simulink model "Demo_MatrixSign_cs"  (Simulink 7.6)
settings: Solver=FixedStepDiscrete  SolverMode=SingleTasking  StartTime=0.0  StopTime=10  FixedStep=1/20  RelTol=1e-3
model workspace (MAT data in the model file):
  mbox_table.block_array(1).src = 'built-in/Subsystem'
  mbox_table.block_array(1).dest = 'Demo_MatrixSign_cs/HighwayOverhang_1'
  mbox_table.block_array(1).mode = 0
  mbox_table.block_array(2).src = 'simulink/Sinks/Out1'
  mbox_table.block_array(2).dest = 'Demo_MatrixSign_cs/HighwayOverhang_1/VISUMatrixSign_HighwayOverhang_1'
  mbox_table.block_array(2).mode = 0
  mbox_table.block_array(3).src = 'PreScanSimulinkLibrary/VisuMatrixSign'
  mbox_table.block_array(3).dest = 'Demo_MatrixSign_cs/VISUMatrixSign_HighwayOverhang_1'
  mbox_table.block_array(3).mode = 0
  mbox_table.block_array(4).src = 'PreScanSimulinkLibrary/MuxMatrixSign'
  mbox_table.block_array(4).dest = 'Demo_MatrixSign_cs/HighwayOverhang_1/VISUMatrixSign_Mux'
  mbox_table.block_array(4).mode = 0
  mbox_table.block_array(5).src = 'simulink/Sources/Constant'
  mbox_table.block_array(5).dest = 'Demo_MatrixSign_cs/HighwayOverhang_1/VISUMatrixSign_Mux/MatrixSign_1_InitialResource'
  mbox_table.block_array(5).mode = 0
  mbox_table.block_array(6).src = 'simulink/Signal Routing/Switch'
  mbox_table.block_array(6).dest = 'Demo_MatrixSign_cs/HighwayOverhang_1/VISUMatrixSign_Mux/MatrixSign_1_Switch'
  mbox_table.block_array(6).mode = 0
  mbox_table.block_array(7).src = 'Demo_MatrixSign_cs/HighwayOverhang_1/VISUMatrixSign_Mux/MatrixSign_1'
  mbox_table.block_array(7).dest = 'Demo_MatrixSign_cs/HighwayOverhang_1/VISUMatrixSign_Mux/MatrixSign_2'
  mbox_table.block_array(7).mode = 0
  mbox_table.block_array(8).src = 'simulink/Sources/Constant'
  mbox_table.block_array(8).dest = 'Demo_MatrixSign_cs/HighwayOverhang_1/VISUMatrixSign_Mux/MatrixSign_2_InitialResource'
  mbox_table.block_array(8).mode = 0
  mbox_table.block_array(9).src = 'simulink/Signal Routing/Switch'
  mbox_table.block_array(9).dest = 'Demo_MatrixSign_cs/HighwayOverhang_1/VISUMatrixSign_Mux/MatrixSign_2_Switch'
  mbox_table.block_array(9).mode = 0
  mbox_table.block_array(10).src = 'Demo_MatrixSign_cs/VISUMatrixSign_HighwayOverhang_1/visu_MatrixSign_1'
  mbox_table.block_array(10).dest = 'Demo_MatrixSign_cs/VISUMatrixSign_HighwayOverhang_1/visu_MatrixSign_2'
  mbox_table.block_array(10).mode = 0
  mbox_table.block_array(11).src = 'built-in/Note'
  mbox_table.block_array(11).dest = 'Demo_MatrixSign_cs/HighwayOverhang_1/Resources     
    | 
    | 1: .\InformationSign\MatrixSign_Speed_50.png: MatrixSign_Speed_50
    | 2: .\InformationSign\MatrixSign_Speed_70.png: MatrixSign_Speed_70
    | 3: .\InformationSign\MatrixSign_Speed_End.png: MatrixSign_Speed_End
    | 4: .\InformationSign\MatrixSign_Empty.png: MatrixSign_Empty'
  mbox_table.block_array(11).mode = 0
  mbox_table.block_array(12).src = 'built-in/Note'
  mbox_table.block_array(12).dest = 'Demo_MatrixSign_cs/HighwayOverhang_1/Resources     '
  mbox_table.block_array(12).mode = 0
  mbox_table.block_array(13).src = 'simulink/Sinks/Out1'
  mbox_table.block_array(13).dest = 'Demo_MatrixSign_cs/HighwayOverhang_1/VISUMatrixSignLights_HighwayOverhang_1'
  mbox_table.block_array(13).mode = 0
  mbox_table.block_array(14).src = 'PreScanSimulinkLibrary/VisuMatrixSignLights'
  mbox_table.block_array(14).dest = 'Demo_MatrixSign_cs/VISUMatrixSignLights_HighwayOverhang_1'
  mbox_table.block_array(14).mode = 0
  mbox_table.block_array(15).src = 'PreScanSimulinkLibrary/MuxMatrixSignLights'
  mbox_table.block_array(15).dest = 'Demo_MatrixSign_cs/HighwayOverhang_1/VISUMatrixSignLights_Mux'
  mbox_table.block_array(15).mode = 0
  mbox_table.block_array(16).src = 'Demo_MatrixSign_cs/HighwayOverhang_1/VISUMatrixSignLights_Mux/MatrixSign_1'
  mbox_table.block_array(16).dest = 'Demo_MatrixSign_cs/HighwayOverhang_1/VISUMatrixSignLights_Mux/MatrixSign_2'
  mbox_table.block_array(16).mode = 0
  mbox_table.block_array(17).src = 'Demo_MatrixSign_cs/VISUMatrixSignLights_HighwayOverhang_1/conv_Orange_1'
  mbox_table.block_array(17).dest = 'Demo_MatrixSign_cs/VISUMatrixSignLights_HighwayOverhang_1/conv_Orange_2'
  mbox_table.block_array(17).mode = 0
  mbox_table.block_array(18).src = 'Demo_MatrixSign_cs/VISUMatrixSignLights_HighwayOverhang_1/visu_MatrixSignLights_1'
  mbox_table.block_array(18).dest = 'Demo_MatrixSign_cs/VISUMatrixSignLights_HighwayOverhang_1/visu_MatrixSignLights_2'
  mbox_table.block_array(18).mode = 0
  mbox_table.block_array(19).src = 'Demo_MatrixSign_cs/VISUMatrixSignLights_HighwayOverhang_1/conv_Orange_1'
  mbox_table.block_array(19).dest = 'Demo_MatrixSign_cs/VISUMatrixSignLights_HighwayOverhang_1/conv_Orange_3'
  mbox_table.block_array(19).mode = 0
  mbox_table.block_array(20).src = 'Demo_MatrixSign_cs/VISUMatrixSignLights_HighwayOverhang_1/visu_MatrixSignLights_1'
  mbox_table.block_array(20).dest = 'Demo_MatrixSign_cs/VISUMatrixSignLights_HighwayOverhang_1/visu_MatrixSignLights_3'
  mbox_table.block_array(20).mode = 0
  mbox_table.block_array(21).src = 'Demo_MatrixSign_cs/VISUMatrixSignLights_HighwayOverhang_1/conv_Orange_1'
  mbox_table.block_array(21).dest = 'Demo_MatrixSign_cs/VISUMatrixSignLights_HighwayOverhang_1/conv_Orange_4'
  mbox_table.block_array(21).mode = 0
  mbox_table.block_array(22).src = 'Demo_MatrixSign_cs/VISUMatrixSignLights_HighwayOverhang_1/visu_MatrixSignLights_1'
  mbox_table.block_array(22).dest = 'Demo_MatrixSign_cs/VISUMatrixSignLights_HighwayOverhang_1/visu_MatrixSignLights_4'
  mbox_table.block_array(22).mode = 0
  mbox_table.block_array(23).src = 'Demo_MatrixSign_cs/VISUMatrixSignLights_HighwayOverhang_1/conv_Orange_1'
  mbox_table.block_array(23).dest = 'Demo_MatrixSign_cs/VISUMatrixSignLights_HighwayOverhang_1/conv_Orange_5'
  mbox_table.block_array(23).mode = 0
  mbox_table.block_array(24).src = 'Demo_MatrixSign_cs/VISUMatrixSignLights_HighwayOverhang_1/visu_MatrixSignLights_1'
  mbox_table.block_array(24).dest = 'Demo_MatrixSign_cs/VISUMatrixSignLights_HighwayOverhang_1/visu_MatrixSignLights_5'
  mbox_table.block_array(24).mode = 0
  mbox_table.block_array(25).src = 'Demo_MatrixSign_cs/VISUMatrixSignLights_HighwayOverhang_1/conv_Orange_1'
  mbox_table.block_array(25).dest = 'Demo_MatrixSign_cs/VISUMatrixSignLights_HighwayOverhang_1/conv_Orange_6'
  mbox_table.block_array(25).mode = 0
  mbox_table.block_array(26).src = 'Demo_MatrixSign_cs/VISUMatrixSignLights_HighwayOverhang_1/visu_MatrixSignLights_1'
  mbox_table.block_array(26).dest = 'Demo_MatrixSign_cs/VISUMatrixSignLights_HighwayOverhang_1/visu_MatrixSignLights_6'
  mbox_table.block_array(26).mode = 0
  mbox_table.block_array(27).src = 'Demo_MatrixSign_cs/VISUMatrixSignLights_HighwayOverhang_1/conv_Orange_1'
  mbox_table.block_array(27).dest = 'Demo_MatrixSign_cs/VISUMatrixSignLights_HighwayOverhang_1/conv_Orange_7'
  mbox_table.block_array(27).mode = 0
  mbox_table.block_array(28).src = 'Demo_MatrixSign_cs/VISUMatrixSignLights_HighwayOverhang_1/visu_MatrixSignLights_1'
  mbox_table.block_array(28).dest = 'Demo_MatrixSign_cs/VISUMatrixSignLights_HighwayOverhang_1/visu_MatrixSignLights_7'
  mbox_table.block_array(28).mode = 0
  mbox_table.block_array(29).src = 'Demo_MatrixSign_cs/VISUMatrixSignLights_HighwayOverhang_1/conv_Orange_1'
  mbox_table.block_array(29).dest = 'Demo_MatrixSign_cs/VISUMatrixSignLights_HighwayOverhang_1/conv_Orange_8'
  mbox_table.block_array(29).mode = 0
  mbox_table.block_array(30).src = 'Demo_MatrixSign_cs/VISUMatrixSignLights_HighwayOverhang_1/visu_MatrixSignLights_1'
  mbox_table.block_array(30).dest = 'Demo_MatrixSign_cs/VISUMatrixSignLights_HighwayOverhang_1/visu_MatrixSignLights_8'
  mbox_table.block_array(30).mode = 0
  mbox_table.block_array(31).src = 'SimCoreLibrary/SimCoreConfiguration'
  mbox_table.block_array(31).dest = 'Demo_MatrixSign_cs/SimCoreConfiguration'
  mbox_table.block_array(31).mode = 0
  mbox_table.block_array(32).src = 'SimCoreLibrary/Actuators'
  mbox_table.block_array(32).dest = 'Demo_MatrixSign_cs/Actuators'
  mbox_table.block_array(32).mode = 0
  mbox_table.block_array(33).src = 'SimCoreLibrary/SetActuators'
  mbox_table.block_array(33).dest = 'Demo_MatrixSign_cs/SetActuators'
  mbox_table.block_array(33).mode = 0
  mbox_table.block_array(34).src = 'SimCoreLibrary/SimCoreInfo'
  mbox_table.block_array(34).dest = 'Demo_MatrixSign_cs/SimCoreInfo'
  mbox_table.block_array(34).mode = 0
  mbox_table.block_array(35).src = 'PreScanSimulinkLibrary/Regenerate'
  mbox_table.block_array(35).dest = 'Demo_MatrixSign_cs/Regenerate'
  mbox_table.block_array(35).mode = 0
  mbox_table.block_array(36).src = 'PreScanSimulinkLibrary/Record for Replay  '
  mbox_table.block_array(36).dest = 'Demo_MatrixSign_cs/Record for Replay  '
  mbox_table.block_array(36).mode = 0
  mbox_table.block_array(37).src = 'PreScanSimulinkLibrary/Open Useful Blocks'
  mbox_table.block_array(37).dest = 'Demo_MatrixSign_cs/Open Useful Blocks'
  mbox_table.block_array(37).mode = 0
  mbox_table.block_array(38).src = 'PreScanSimulinkLibrary/PreScan Options   '
  mbox_table.block_array(38).dest = 'Demo_MatrixSign_cs/PreScan Options   '
  mbox_table.block_array(38).mode = 0
  mbox_table.block_array(39).src = 'built-in/Note'
  mbox_table.block_array(39).dest = 'Demo_MatrixSign_cs/Version:                  '
  mbox_table.block_array(39).mode = 0
  mbox_table.block_array(40).src = 'built-in/Note'
  mbox_table.block_array(40).dest = 'Demo_MatrixSign_cs/7.4.0'
  mbox_table.block_array(40).mode = 0
  mbox_table.block_array(41).src = 'built-in/Note'
  mbox_table.block_array(41).dest = 'Demo_MatrixSign_cs/Author(s):                '
  mbox_table.block_array(41).mode = 0
  mbox_table.block_array(42).src = 'built-in/Note'
  mbox_table.block_array(42).dest = 'Demo_MatrixSign_cs/F.J.W. Leneman, (c) TNO 2008'
  mbox_table.block_array(42).mode = 0
  mbox_table.block_array(43).src = 'built-in/Note'
  mbox_table.block_array(43).dest = 'Demo_MatrixSign_cs/Descriptive text:      '
  mbox_table.block_array(43).mode = 0
  mbox_table.block_array(44).src = 'built-in/Note'
  mbox_table.block_array(44).dest = 'Demo_MatrixSign_cs/Demo MatrixSign
    | The demo illustrates the use of
    | the Matrix Sign.
    | 
    | Key-elements:
    | - Matrix Sign
    | - Overhang
    | - Signal Builder Block'
  mbox_table.block_array(44).mode = 0
  mbox_table.block_array(45).src = 'built-in/Note'
  mbox_table.block_array(45).dest = 'Demo_MatrixSign_cs/ID
    | 
    | 1'
  mbox_table.block_array(45).mode = 0
  mbox_table.block_array(46).src = 'built-in/Note'
  mbox_table.block_array(46).dest = 'Demo_MatrixSign_cs/OBU-Beacon ID
    | 
    | '
  mbox_table.block_array(46).mode = 0
  mbox_table.block_array(47).src = 'built-in/Note'
  mbox_table.block_array(47).dest = 'Demo_MatrixSign_cs/TypeID
    | 
    | 15'
  mbox_table.block_array(47).mode = 0
  mbox_table.block_array(48).src = 'built-in/Note'
  mbox_table.block_array(48).dest = 'Demo_MatrixSign_cs/TypeTag
    | 
    | Anim traffic sign'
  mbox_table.block_array(48).mode = 0
  mbox_table.block_array(49).src = 'built-in/Note'
  mbox_table.block_array(49).dest = 'Demo_MatrixSign_cs/SD
    | 
    | Y'
  mbox_table.block_array(49).mode = 0
  mbox_table.block_array(50).src = 'built-in/Note'
  mbox_table.block_array(50).dest = 'Demo_MatrixSign_cs/CD
    | 
    | N'
  mbox_table.block_array(50).mode = 0
  mbox_table.block_array(51).src = 'built-in/Note'
  mbox_table.block_array(51).dest = 'Demo_MatrixSign_cs/Name
    | 
    | HighwayOverhang_1'
  mbox_table.block_array(51).mode = 0
  mbox_table.block_array(52).src = 'built-in/Note'
  mbox_table.block_array(52).dest = 'Demo_MatrixSign_cs/Num ID       OBU-Beacon ID     Type ID      Type Tag             SD        CD             Name                          '
  mbox_table.block_array(52).mode = 0
  mbox_table.block_array(53).src = 'built-in/Terminator'
  mbox_table.block_array(53).dest = 'Demo_MatrixSign_cs/Terminator_1'
  mbox_table.block_array(53).mode = 1
  mbox_table.block_index : java.util.Hashtable (value not decoded)
  mbox_table.line_array(1).sys = 'Demo_MatrixSign_cs/HighwayOverhang_1'
  mbox_table.line_array(1).line_id = 'L1'
  mbox_table.line_array(1).iport = 'VISUMatrixSign_HighwayOverhang_1/1'
  mbox_table.line_array(1).oport = 'VISUMatrixSign_Mux/1'
  mbox_table.line_array(1).mode = 0
  mbox_table.line_array(2).sys = 'Demo_MatrixSign_cs'
  mbox_table.line_array(2).line_id = 'L2'
  mbox_table.line_array(2).iport = 'VISUMatrixSign_HighwayOverhang_1/1'
  mbox_table.line_array(2).oport = 'HighwayOverhang_1/1'
  mbox_table.line_array(2).mode = 0
  mbox_table.line_array(3).sys = 'Demo_MatrixSign_cs/HighwayOverhang_1/VISUMatrixSign_Mux'
  mbox_table.line_array(3).line_id = 'L4'
  mbox_table.line_array(3).iport = 'MatrixSign_1_Switch/1'
  mbox_table.line_array(3).oport = 'MatrixSign_1/1'
  mbox_table.line_array(3).mode = 0
  mbox_table.line_array(4).sys = 'Demo_MatrixSign_cs/HighwayOverhang_1/VISUMatrixSign_Mux'
  mbox_table.line_array(4).line_id = 'L4'
  mbox_table.line_array(4).iport = 'MatrixSign_1_Switch/2'
  mbox_table.line_array(4).oport = 'MatrixSign_1/1'
  mbox_table.line_array(4).mode = 0
  mbox_table.line_array(5).sys = 'Demo_MatrixSign_cs/HighwayOverhang_1/VISUMatrixSign_Mux'
  mbox_table.line_array(5).line_id = 'L5'
  mbox_table.line_array(5).iport = 'MatrixSign_1_Switch/3'
  mbox_table.line_array(5).oport = 'MatrixSign_1_InitialResource/1'
  mbox_table.line_array(5).mode = 0
  mbox_table.line_array(6).sys = 'Demo_MatrixSign_cs/HighwayOverhang_1/VISUMatrixSign_Mux'
  mbox_table.line_array(6).line_id = 'L6'
  mbox_table.line_array(6).iport = 'SubMuxMatrixSign/1'
  mbox_table.line_array(6).oport = 'MatrixSign_1_Switch/1'
  mbox_table.line_array(6).mode = 0
  mbox_table.line_array(7).sys = 'Demo_MatrixSign_cs/HighwayOverhang_1/VISUMatrixSign_Mux'
  mbox_table.line_array(7).line_id = 'L8'
  mbox_table.line_array(7).iport = 'MatrixSign_2_Switch/1'
  mbox_table.line_array(7).oport = 'MatrixSign_2/1'
  mbox_table.line_array(7).mode = 0
  mbox_table.line_array(8).sys = 'Demo_MatrixSign_cs/HighwayOverhang_1/VISUMatrixSign_Mux'
  mbox_table.line_array(8).line_id = 'L8'
  mbox_table.line_array(8).iport = 'MatrixSign_2_Switch/2'
  mbox_table.line_array(8).oport = 'MatrixSign_2/1'
  mbox_table.line_array(8).mode = 0
  mbox_table.line_array(9).sys = 'Demo_MatrixSign_cs/HighwayOverhang_1/VISUMatrixSign_Mux'
  mbox_table.line_array(9).line_id = 'L9'
  mbox_table.line_array(9).iport = 'MatrixSign_2_Switch/3'
  mbox_table.line_array(9).oport = 'MatrixSign_2_InitialResource/1'
  mbox_table.line_array(9).mode = 0
  mbox_table.line_array(10).sys = 'Demo_MatrixSign_cs/HighwayOverhang_1/VISUMatrixSign_Mux'
  mbox_table.line_array(10).line_id = 'L10'
  mbox_table.line_array(10).iport = 'SubMuxMatrixSign/2'
  mbox_table.line_array(10).oport = 'MatrixSign_2_Switch/1'
  mbox_table.line_array(10).mode = 0
  mbox_table.line_array(11).sys = 'Demo_MatrixSign_cs/VISUMatrixSign_HighwayOverhang_1'
  mbox_table.line_array(11).line_id = 'L11'
  mbox_table.line_array(11).iport = 'visu_MatrixSign_2/1'
  mbox_table.line_array(11).oport = 'SubMuxVisuMatrixSign/2'
  mbox_table.line_array(11).mode = 0
  mbox_table.line_array(12).sys = 'Demo_MatrixSign_cs/HighwayOverhang_1'
  mbox_table.line_array(12).line_id = 'L12'
  mbox_table.line_array(12).iport = 'VISUMatrixSignLights_HighwayOverhang_1/1'
  mbox_table.line_array(12).oport = 'VISUMatrixSignLights_Mux/1'
  mbox_table.line_array(12).mode = 0
  mbox_table.line_array(13).sys = 'Demo_MatrixSign_cs'
  mbox_table.line_array(13).line_id = 'L13'
  mbox_table.line_array(13).iport = 'VISUMatrixSignLights_HighwayOverhang_1/1'
  mbox_table.line_array(13).oport = 'HighwayOverhang_1/2'
  mbox_table.line_array(13).mode = 0
  mbox_table.line_array(14).sys = 'Demo_MatrixSign_cs/HighwayOverhang_1/VISUMatrixSignLights_Mux'
  mbox_table.line_array(14).line_id = 'L14'
  mbox_table.line_array(14).iport = 'SubMuxMatrixSignLights/2'
  mbox_table.line_array(14).oport = 'MatrixSign_2/1'
  mbox_table.line_array(14).mode = 0
  mbox_table.line_array(15).sys = 'Demo_MatrixSign_cs/VISUMatrixSignLights_HighwayOverhang_1'
  mbox_table.line_array(15).line_id = 'L15'
  mbox_table.line_array(15).iport = 'conv_Orange_2/1'
  mbox_table.line_array(15).oport = 'SubMuxVisuMatrixSignLights/2'
  mbox_table.line_array(15).mode = 0
  mbox_table.line_array(16).sys = 'Demo_MatrixSign_cs/VISUMatrixSignLights_HighwayOverhang_1'
  mbox_table.line_array(16).line_id = 'L16'
  mbox_table.line_array(16).iport = 'visu_MatrixSignLights_2/1'
  mbox_table.line_array(16).oport = 'conv_Orange_2/1'
  mbox_table.line_array(16).mode = 0
  mbox_table.line_array(17).sys = 'Demo_MatrixSign_cs/VISUMatrixSignLights_HighwayOverhang_1'
  mbox_table.line_array(17).line_id = 'L17'
  mbox_table.line_array(17).iport = 'conv_Orange_3/1'
  mbox_table.line_array(17).oport = 'SubMuxVisuMatrixSignLights/3'
  mbox_table.line_array(17).mode = 0
  mbox_table.line_array(18).sys = 'Demo_MatrixSign_cs/VISUMatrixSignLights_HighwayOverhang_1'
  mbox_table.line_array(18).line_id = 'L18'
  mbox_table.line_array(18).iport = 'visu_MatrixSignLights_3/1'
  mbox_table.line_array(18).oport = 'conv_Orange_3/1'
  mbox_table.line_array(18).mode = 0
  mbox_table.line_array(19).sys = 'Demo_MatrixSign_cs/VISUMatrixSignLights_HighwayOverhang_1'
  mbox_table.line_array(19).line_id = 'L19'
  mbox_table.line_array(19).iport = 'conv_Orange_4/1'
  mbox_table.line_array(19).oport = 'SubMuxVisuMatrixSignLights/4'
  mbox_table.line_array(19).mode = 0
  mbox_table.line_array(20).sys = 'Demo_MatrixSign_cs/VISUMatrixSignLights_HighwayOverhang_1'
  mbox_table.line_array(20).line_id = 'L20'
  mbox_table.line_array(20).iport = 'visu_MatrixSignLights_4/1'
  mbox_table.line_array(20).oport = 'conv_Orange_4/1'
  mbox_table.line_array(20).mode = 0
  mbox_table.line_array(21).sys = 'Demo_MatrixSign_cs/VISUMatrixSignLights_HighwayOverhang_1'
  mbox_table.line_array(21).line_id = 'L21'
  mbox_table.line_array(21).iport = 'conv_Orange_5/1'
  mbox_table.line_array(21).oport = 'SubMuxVisuMatrixSignLights/5'
  mbox_table.line_array(21).mode = 0
  mbox_table.line_array(22).sys = 'Demo_MatrixSign_cs/VISUMatrixSignLights_HighwayOverhang_1'
  mbox_table.line_array(22).line_id = 'L22'
  mbox_table.line_array(22).iport = 'visu_MatrixSignLights_5/1'
  mbox_table.line_array(22).oport = 'conv_Orange_5/1'
  mbox_table.line_array(22).mode = 0
  mbox_table.line_array(23).sys = 'Demo_MatrixSign_cs/VISUMatrixSignLights_HighwayOverhang_1'
  mbox_table.line_array(23).line_id = 'L23'
  mbox_table.line_array(23).iport = 'conv_Orange_6/1'
  mbox_table.line_array(23).oport = 'SubMuxVisuMatrixSignLights/6'
  mbox_table.line_array(23).mode = 0
  mbox_table.line_array(24).sys = 'Demo_MatrixSign_cs/VISUMatrixSignLights_HighwayOverhang_1'
  mbox_table.line_array(24).line_id = 'L24'
  mbox_table.line_array(24).iport = 'visu_MatrixSignLights_6/1'
  mbox_table.line_array(24).oport = 'conv_Orange_6/1'
  mbox_table.line_array(24).mode = 0
  mbox_table.line_array(25).sys = 'Demo_MatrixSign_cs/VISUMatrixSignLights_HighwayOverhang_1'
  mbox_table.line_array(25).line_id = 'L25'
  mbox_table.line_array(25).iport = 'conv_Orange_7/1'
  mbox_table.line_array(25).oport = 'SubMuxVisuMatrixSignLights/7'
  mbox_table.line_array(25).mode = 0
  mbox_table.line_array(26).sys = 'Demo_MatrixSign_cs/VISUMatrixSignLights_HighwayOverhang_1'
  mbox_table.line_array(26).line_id = 'L26'
  mbox_table.line_array(26).iport = 'visu_MatrixSignLights_7/1'
  mbox_table.line_array(26).oport = 'conv_Orange_7/1'
  mbox_table.line_array(26).mode = 0
  mbox_table.line_array(27).sys = 'Demo_MatrixSign_cs/VISUMatrixSignLights_HighwayOverhang_1'
  mbox_table.line_array(27).line_id = 'L27'
  mbox_table.line_array(27).iport = 'conv_Orange_8/1'
  mbox_table.line_array(27).oport = 'SubMuxVisuMatrixSignLights/8'
  mbox_table.line_array(27).mode = 0
  mbox_table.line_array(28).sys = 'Demo_MatrixSign_cs/VISUMatrixSignLights_HighwayOverhang_1'
  mbox_table.line_array(28).line_id = 'L28'
  mbox_table.line_array(28).iport = 'visu_MatrixSignLights_8/1'
  mbox_table.line_array(28).oport = 'conv_Orange_8/1'
  mbox_table.line_array(28).mode = 0
  mbox_table.line_array(29).sys = 'Demo_MatrixSign_cs'
  mbox_table.line_array(29).line_id = 'l1'
  mbox_table.line_array(29).iport = 'Terminator_1/1'
  mbox_table.line_array(29).oport = 'SetActuators/1'
  mbox_table.line_array(29).mode = 1
  mbox_table.line_index : java.util.Hashtable (value not decoded)
  mbox_table.next_linenr = 29
  mbox_table.next_termlinenr = 2
  model_closed = 0
  sim_status = 0
PreLoadFcn:
  | check_NUTS_defined
  | model_closed = 0;
  | assignin('base',['model_closed_' bdroot],false);
InitFcn:
  | PreScanExperimentInitFcn(bdroot)
StopFcn:
  | PreScanExperimentStopFcn(bdroot)
undefined symbols (not defined in the file): sigbuilder_block
CloseFcn:
  | evalin('base',['clear model_closed_' bdroot]);
  | model_closed = 1;
settings Model: Creator=PRESCAN  LastModifiedBy=buildbot
settings OptimizationCC: InitFltsAndDblsToZero=on
settings DebuggingCC: SaveWithParameterizedLinksMsg=none  SignalResolutionControl=TryResolveAllWithWarning  MultiTaskDSMMsg=warning  MultiTaskCondExecSysMsg=none
settings RTWCC: IncludeERTFirstTime=on
settings GRTTargetCC: TargetFcnLib=ansi_tfl_tmw.mat

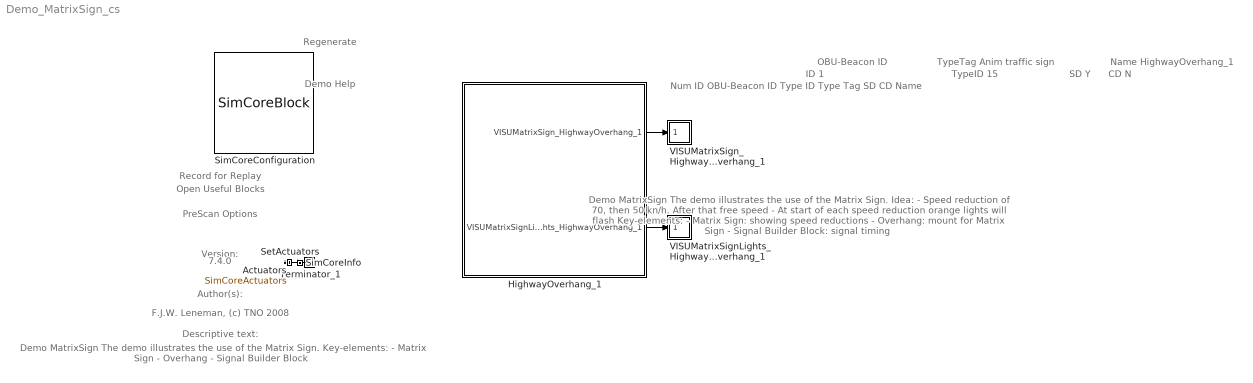
== system Demo_MatrixSign_cs ==
  note: Demo MatrixSign
      | The demo illustrates the use of the Matrix Sign.
      |
      | Idea:
      | - Speed reduction of 70, then 50 kn/h. After that free speed
      | - At start of each speed reduction orange lights will flash
      |
      | Key-elements:
      | - Matrix Sign: showing speed reductions
      | - Overhang: mount for Matrix Sign
      | - Signal Builder Block: signal timing
  note: Demo Help
  note: Regenerate
  note: Record for Replay
  note: Open Useful Blocks
  note: PreScan Options
  note: Version:
  note: 7.4.0
  note: Author(s):
  note: F.J.W. Leneman, (c) TNO 2008
  note: Descriptive text:
  note: Demo MatrixSign
      | The demo illustrates the use of
      | the Matrix Sign.
      |
      | Key-elements:
      | - Matrix Sign
      | - Overhang
      | - Signal Builder Block
  note: ID
      |
      | 1
  note: OBU-Beacon ID
  note: TypeID
      |
      | 15
  note: TypeTag
      |
      | Anim traffic sign
  note: SD
      |
      | Y
  note: CD
      |
      | N
  note: Name
      |
      | HighwayOverhang_1
  note: Num ID OBU-Beacon ID Type ID Type Tag SD CD Name
  Actuators : DataStoreMemory  Tag=Actuators  DataStoreName=SimCoreActuators  InitialValue=zeros(130,1)
      settings: DeleteFcn=PreScanBlockDeleteFcn;
  HighwayOverhang_1 : Subsystem  Tag=WorldObjectSubSystem  InitFcn=|
      | UniqueId = '10';
      | UniqueId = '26';
      mask Display: image(imread('HighwayOverhang.jpg'));color('white');text(0,0,' ID=1\n')
  SetActuators : Subsystem  Tag=SetActuators  Priority=1  mask(PreScan Simulation Core Block){TimeStep=1/20, NrOfActuators=130}
      mask prompts: TimeStep "Timestep [s]"; NrOfActuators "Number of actuator values"
      mask help:
      | Please do not remove this block from the PreScan compilation sheet,
      | as it contains essential configuration parameters for a PreScan simulation.
      settings: DeleteFcn=PreScanBlockDeleteFcn;
  SimCoreConfiguration : M-S-Function  Tag=SimCoreConfiguration  Description=10204DA34D8ECD0E2F4201D869486A065A9BB0BDE78EC91E8B3E87CEDEA871F6  FunctionName=SimCoreBlock  Parameters=ExperimentXML PortsXML SimulationCore HostName CheckStart EnableLog RfR EnableGPUAccel ShowComputationTime  mask(PreScan Simulation Core Configurator){SimulationCore=NUTS, HostName=0, CheckStart=0, prescanversion='7.4.0', EnableLog=off, RfR=0, EnableGPUAccel=off, ShowComputationTime=off}
      mask prompts: SimulationCore "Simulation Core"; HostName "Simulation Host"; CheckStart "Show START Dialog"; prescanversion "PreScan Version"; EnableLog "Create TA Log"; RfR "Record for Replay"; EnableGPUAccel "Enable GPU Acceleration"; ShowComputationTime "Show ComputationTime Scope"
      mask help:
      | Please do not remove this block from the PreScan compilation sheet,
      | as it contains essential configuration parameter for a PreScan simulation.
      mask init:
      | model = bdroot;
      | ExperimentXML = [model(1:end-3) '.pex'];
      | PortsXML = [model '_ports.pcd'];
      settings: DeleteFcn=PreScanBlockDeleteFcn;  ModelCloseFcn=assignin('base',['model_closed_' bdroot],true);
      mask Help: eval('openHelp(812)')
      mask Display: image(imread('prescanlogo.ico'))
  SimCoreInfo : Subsystem  Tag=SimCoreInfo
  Terminator_1 : Terminator
  VISUMatrixSignLights_HighwayOverhang_1 : Subsystem  Tag=VisuMatrixSignLights  Priority=0
      settings: DeleteFcn=PreScanBlockDeleteFcn;
      mask Type: PreScan Sink Block: VisuMatrixSign
      mask Description:
      | The VisuMatrixSign block provides a way to adapt the texture of the plates connected to an overhang, based on Resource IDs of the texture files.
      | 
      | For more information, please click Help.
      mask Help: eval('openHelp()')
      mask Display: image(imread('HighwaySpeedMatrix.png'))
  VISUMatrixSign_HighwayOverhang_1 : Subsystem  Tag=VisuMatrixSign  Priority=0
      settings: DeleteFcn=PreScanBlockDeleteFcn;
      mask Type: PreScan Sink Block: VisuMatrixSign
      mask Description:
      | The VisuMatrixSign block provides a way to adapt the texture of the plates connected to an overhang, based on Resource IDs of the texture files.
      | 
      | For more information, please click Help.
      mask Help: eval('openHelp()')
      mask Display: image(imread('HighwaySpeedMatrix.png'))
  wires:
  HighwayOverhang_1/1(VISUMatrixSign_HighwayOverhang_1) -> VISUMatrixSign_HighwayOverhang_1/1(MatrixSigns)
  HighwayOverhang_1/2(VISUMatrixSignLights_HighwayOverhang_1) -> VISUMatrixSignLights_HighwayOverhang_1/1(MatrixSignLights)
  SetActuators/1(dummy) -> Terminator_1/1

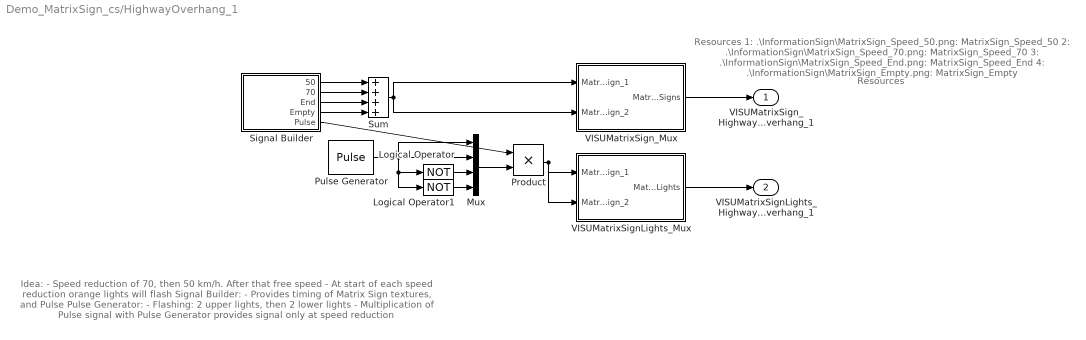
== system Demo_MatrixSign_cs/HighwayOverhang_1 ==
  note: Idea:
      | - Speed reduction of 70, then 50 km/h. After that free speed
      | - At start of each speed reduction orange lights will flash
      |
      | Signal Builder:
      | - Provides timing of Matrix Sign textures, and Pulse
      |
      | Pulse Generator:
      | - Flashing: 2 upper lights, then 2 lower lights
      | - Multiplication of Pulse signal with Pulse Generator provides
      |   signal only at speed reduction
  note: Resources
      |
      | 1: .\InformationSign\MatrixSign_Speed_50.png: MatrixSign_Speed_50
      | 2: .\InformationSign\MatrixSign_Speed_70.png: MatrixSign_Speed_70
      | 3: .\InformationSign\MatrixSign_Speed_End.png: MatrixSign_Speed_End
      | 4: .\InformationSign\MatrixSign_Empty.png: MatrixSign_Empty
  note: Resources
  Logical Operator : Logic  Operator=NOT  AllPortsSameDT=off  OutDataTypeStr=float('double')
  Logical Operator1 : Logic  Operator=NOT  AllPortsSameDT=off  OutDataTypeStr=float('double')
  Mux : Mux
  Product : Product  RndMeth=Zero
  Pulse Generator : DiscretePulseGenerator  PulseType=Time based  Period=0.2  PulseWidth=50
  Signal Builder : Subsystem  Tag=STV Subsys  LoadFcn=sigbuilder_block('load');  StartFcn=sigbuilder_block('start');  StopFcn=sigbuilder_block('stop');  ClipboardFcn=sigbuilder_block('clipboard');  mask(Sigbuilder block){}
      mask help: Sigbuilder GUI
      mask init:
      | if ~strcmp(get_param(bdroot(gcbh),'SimulationStatus'),'stopped') tuvar = sigbuilder_block('maskInit'); end
      settings: CopyFcn=sigbuilder_block('copy');  DeleteFcn=sigbuilder_block('delete');  ModelCloseFcn=sigbuilder_block('modelClose');  PreSaveFcn=sigbuilder_block('preSave');  NameChangeFcn=sigbuilder_block('namechange');  OpenFcn=sigbuilder_block('open',[123 249 550.5 399.75 ]);  CloseFcn=sigbuilder_block('close');
      mask Display: plot(0,0,100,100,[10,10,40,40,10],[80,20,20,80,80],[40,10],[50,50], [40,27,10],[65,72,56],[40,25,25,10],[28,28,43,43]);
  Sum : Sum  Inputs=++++
  VISUMatrixSignLights_Mux : Subsystem  Tag=MuxMatrixSignLights
      settings: DeleteFcn=PreScanBlockDeleteFcn;
      mask Type: PreScan Mux Block:
  VISUMatrixSign_Mux : Subsystem  Tag=MuxMatrixSign
      settings: DeleteFcn=PreScanBlockDeleteFcn;
      mask Type: PreScan Mux Block:
  VISUMatrixSign_HighwayOverhang_1 : Outport  Tag=VisuMatrixSignOutport  SampleTime=1/20
  VISUMatrixSignLights_HighwayOverhang_1 : Outport  Tag=VisuMatrixSignLightsOutport  Port=2  SampleTime=1/20
  wires:
  Logical Operator/1 -> Mux/3
  Logical Operator1/1 -> Mux/4
  Pulse Generator/1 -> Mux/1, Mux/2, Logical Operator/1, Logical Operator1/1
  Mux/1 -> Product/2
  VISUMatrixSign_Mux/1(MatrixSigns) -> VISUMatrixSign_HighwayOverhang_1/1
  VISUMatrixSignLights_Mux/1(MatrixSignLights) -> VISUMatrixSignLights_HighwayOverhang_1/1
  Sum/1 -> VISUMatrixSign_Mux/1(MatrixSign_1), VISUMatrixSign_Mux/2(MatrixSign_2)
  Product/1 -> VISUMatrixSignLights_Mux/1(MatrixSign_1), VISUMatrixSignLights_Mux/2(MatrixSign_2)
  Signal Builder/4(Empty) -> Sum/4
  Signal Builder/3(End) -> Sum/3
  Signal Builder/2(70) -> Sum/2
  Signal Builder/1(50) -> Sum/1
  Signal Builder/5(Pulse) -> Product/1

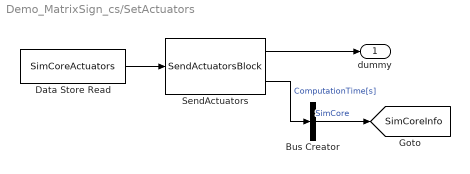
== system Demo_MatrixSign_cs/SetActuators ==
  Bus Creator : BusCreator  Inputs=1
  Data Store Read : DataStoreRead  DataStoreName=SimCoreActuators  SampleTime=TimeStep
  SendActuators : M-S-Function  FunctionName=SendActuatorsBlock  Parameters=TimeStep NrOfActuators
  dummy : Outport
  tag scope: SimCoreInfo=global
  wires:
  Bus Creator/1 -> [SimCoreInfo]  "SimCore"
  SendActuators/2 -> Bus Creator/1  "ComputationTime[s]"
  SendActuators/1 -> dummy/1
  Data Store Read/1 -> SendActuators/1

== system Demo_MatrixSign_cs/SimCoreInfo ==
  Bus Selector : BusSelector  OutputSignals=ComputationTime[s]
  Time : Scope
      settings: TimeRange=10  YMin=0  YMax=0.5  SaveName=ComputationTime
  wires:
  Bus Selector/1 -> Time/1  "<ComputationTime[s]>"
  [SimCoreInfo] -> Bus Selector/1

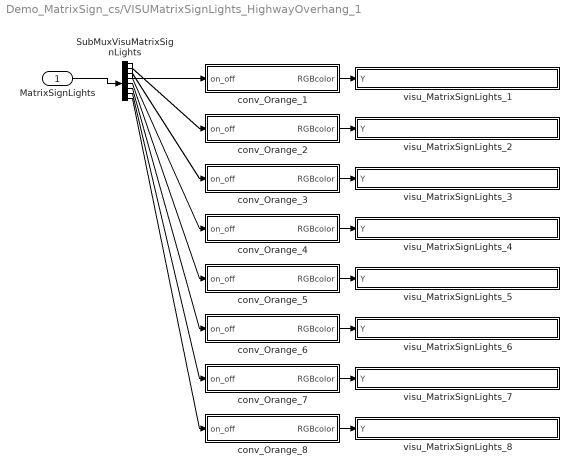
== system Demo_MatrixSign_cs/VISUMatrixSignLights_HighwayOverhang_1 ==
  MatrixSignLights : Inport
  SubMuxVisuMatrixSignLights : Demux  Outputs=8
  conv_Orange_1 : Subsystem
  conv_Orange_2 : Subsystem
  conv_Orange_3 : Subsystem
  conv_Orange_4 : Subsystem
  conv_Orange_5 : Subsystem
  conv_Orange_6 : Subsystem
  conv_Orange_7 : Subsystem
  conv_Orange_8 : Subsystem
  visu_MatrixSignLights_1 : Subsystem  mask(ToSensorWorld){PortName=MatrixSign_1_Light_1, PortIndex=2, PortWidth=16, TimeStep=1/20}
      mask prompts: PortName "Port Name [-]"; PortIndex "Index [-]"; PortWidth "Port Dimensions [-]"; TimeStep "Upload Period [s]"
      mask help: Sends signal(s) from Simulink to the Sensor World
      mask Help:
      | Sends signal(s) from Simulink to the Sensor World.
      | 
      | - Port Name [-]: specifies the name of the output terminal of the Simulink block.
      | - Index [-]: specifies the start position in the output vector sent to the Sensor World
      | - Port dimensions [-]: specifies the width (number of scalars) of the output port
      | - Upload period [s]: specifies the upload period (in seconds) of the port.
      mask Display: port_label('input', 1, PortName)
  visu_MatrixSignLights_2 : Subsystem  mask(ToSensorWorld){PortName=MatrixSign_1_Light_2, PortIndex=18, PortWidth=16, TimeStep=1/20}
      mask prompts: PortName "Port Name [-]"; PortIndex "Index [-]"; PortWidth "Port Dimensions [-]"; TimeStep "Upload Period [s]"
      mask help: Sends signal(s) from Simulink to the Sensor World
      mask Help:
      | Sends signal(s) from Simulink to the Sensor World.
      | 
      | - Port Name [-]: specifies the name of the output terminal of the Simulink block.
      | - Index [-]: specifies the start position in the output vector sent to the Sensor World
      | - Port dimensions [-]: specifies the width (number of scalars) of the output port
      | - Upload period [s]: specifies the upload period (in seconds) of the port.
      mask Display: port_label('input', 1, PortName)
  visu_MatrixSignLights_3 : Subsystem  mask(ToSensorWorld){PortName=MatrixSign_1_Light_3, PortIndex=34, PortWidth=16, TimeStep=1/20}
      mask prompts: PortName "Port Name [-]"; PortIndex "Index [-]"; PortWidth "Port Dimensions [-]"; TimeStep "Upload Period [s]"
      mask help: Sends signal(s) from Simulink to the Sensor World
      mask Help:
      | Sends signal(s) from Simulink to the Sensor World.
      | 
      | - Port Name [-]: specifies the name of the output terminal of the Simulink block.
      | - Index [-]: specifies the start position in the output vector sent to the Sensor World
      | - Port dimensions [-]: specifies the width (number of scalars) of the output port
      | - Upload period [s]: specifies the upload period (in seconds) of the port.
      mask Display: port_label('input', 1, PortName)
  visu_MatrixSignLights_4 : Subsystem  mask(ToSensorWorld){PortName=MatrixSign_1_Light_4, PortIndex=50, PortWidth=16, TimeStep=1/20}
      mask prompts: PortName "Port Name [-]"; PortIndex "Index [-]"; PortWidth "Port Dimensions [-]"; TimeStep "Upload Period [s]"
      mask help: Sends signal(s) from Simulink to the Sensor World
      mask Help:
      | Sends signal(s) from Simulink to the Sensor World.
      | 
      | - Port Name [-]: specifies the name of the output terminal of the Simulink block.
      | - Index [-]: specifies the start position in the output vector sent to the Sensor World
      | - Port dimensions [-]: specifies the width (number of scalars) of the output port
      | - Upload period [s]: specifies the upload period (in seconds) of the port.
      mask Display: port_label('input', 1, PortName)
  visu_MatrixSignLights_5 : Subsystem  mask(ToSensorWorld){PortName=MatrixSign_2_Light_1, PortIndex=66, PortWidth=16, TimeStep=1/20}
      mask prompts: PortName "Port Name [-]"; PortIndex "Index [-]"; PortWidth "Port Dimensions [-]"; TimeStep "Upload Period [s]"
      mask help: Sends signal(s) from Simulink to the Sensor World
      mask Help:
      | Sends signal(s) from Simulink to the Sensor World.
      | 
      | - Port Name [-]: specifies the name of the output terminal of the Simulink block.
      | - Index [-]: specifies the start position in the output vector sent to the Sensor World
      | - Port dimensions [-]: specifies the width (number of scalars) of the output port
      | - Upload period [s]: specifies the upload period (in seconds) of the port.
      mask Display: port_label('input', 1, PortName)
  visu_MatrixSignLights_6 : Subsystem  mask(ToSensorWorld){PortName=MatrixSign_2_Light_2, PortIndex=82, PortWidth=16, TimeStep=1/20}
      mask prompts: PortName "Port Name [-]"; PortIndex "Index [-]"; PortWidth "Port Dimensions [-]"; TimeStep "Upload Period [s]"
      mask help: Sends signal(s) from Simulink to the Sensor World
      mask Help:
      | Sends signal(s) from Simulink to the Sensor World.
      | 
      | - Port Name [-]: specifies the name of the output terminal of the Simulink block.
      | - Index [-]: specifies the start position in the output vector sent to the Sensor World
      | - Port dimensions [-]: specifies the width (number of scalars) of the output port
      | - Upload period [s]: specifies the upload period (in seconds) of the port.
      mask Display: port_label('input', 1, PortName)
  visu_MatrixSignLights_7 : Subsystem  mask(ToSensorWorld){PortName=MatrixSign_2_Light_3, PortIndex=98, PortWidth=16, TimeStep=1/20}
      mask prompts: PortName "Port Name [-]"; PortIndex "Index [-]"; PortWidth "Port Dimensions [-]"; TimeStep "Upload Period [s]"
      mask help: Sends signal(s) from Simulink to the Sensor World
      mask Help:
      | Sends signal(s) from Simulink to the Sensor World.
      | 
      | - Port Name [-]: specifies the name of the output terminal of the Simulink block.
      | - Index [-]: specifies the start position in the output vector sent to the Sensor World
      | - Port dimensions [-]: specifies the width (number of scalars) of the output port
      | - Upload period [s]: specifies the upload period (in seconds) of the port.
      mask Display: port_label('input', 1, PortName)
  visu_MatrixSignLights_8 : Subsystem  mask(ToSensorWorld){PortName=MatrixSign_2_Light_4, PortIndex=114, PortWidth=16, TimeStep=1/20}
      mask prompts: PortName "Port Name [-]"; PortIndex "Index [-]"; PortWidth "Port Dimensions [-]"; TimeStep "Upload Period [s]"
      mask help: Sends signal(s) from Simulink to the Sensor World
      mask Help:
      | Sends signal(s) from Simulink to the Sensor World.
      | 
      | - Port Name [-]: specifies the name of the output terminal of the Simulink block.
      | - Index [-]: specifies the start position in the output vector sent to the Sensor World
      | - Port dimensions [-]: specifies the width (number of scalars) of the output port
      | - Upload period [s]: specifies the upload period (in seconds) of the port.
      mask Display: port_label('input', 1, PortName)
  wires:
  conv_Orange_1/1(RGBcolor) -> visu_MatrixSignLights_1/1(Y)
  MatrixSignLights/1 -> SubMuxVisuMatrixSignLights/1
  SubMuxVisuMatrixSignLights/1 -> conv_Orange_1/1(on_off)
  SubMuxVisuMatrixSignLights/2 -> conv_Orange_2/1(on_off)
  conv_Orange_2/1(RGBcolor) -> visu_MatrixSignLights_2/1(Y)
  SubMuxVisuMatrixSignLights/3 -> conv_Orange_3/1(on_off)
  conv_Orange_3/1(RGBcolor) -> visu_MatrixSignLights_3/1(Y)
  SubMuxVisuMatrixSignLights/4 -> conv_Orange_4/1(on_off)
  conv_Orange_4/1(RGBcolor) -> visu_MatrixSignLights_4/1(Y)
  SubMuxVisuMatrixSignLights/5 -> conv_Orange_5/1(on_off)
  conv_Orange_5/1(RGBcolor) -> visu_MatrixSignLights_5/1(Y)
  SubMuxVisuMatrixSignLights/6 -> conv_Orange_6/1(on_off)
  conv_Orange_6/1(RGBcolor) -> visu_MatrixSignLights_6/1(Y)
  SubMuxVisuMatrixSignLights/7 -> conv_Orange_7/1(on_off)
  conv_Orange_7/1(RGBcolor) -> visu_MatrixSignLights_7/1(Y)
  SubMuxVisuMatrixSignLights/8 -> conv_Orange_8/1(on_off)
  conv_Orange_8/1(RGBcolor) -> visu_MatrixSignLights_8/1(Y)

== system Demo_MatrixSign_cs/VISUMatrixSign_HighwayOverhang_1 ==
  MatrixSigns : Inport
  SubMuxVisuMatrixSign : Demux  Outputs=2
  visu_MatrixSign_1 : Subsystem  mask(ToSensorWorld){PortName=MatrixSign_1, PortIndex=0, PortWidth=1, TimeStep=1/20}
      mask prompts: PortName "Port Name [-]"; PortIndex "Index [-]"; PortWidth "Port Dimensions [-]"; TimeStep "Upload Period [s]"
      mask help: Sends signal(s) from Simulink to the Sensor World
      mask Help:
      | Sends signal(s) from Simulink to the Sensor World.
      | 
      | - Port Name [-]: specifies the name of the output terminal of the Simulink block.
      | - Index [-]: specifies the start position in the output vector sent to the Sensor World
      | - Port dimensions [-]: specifies the width (number of scalars) of the output port
      | - Upload period [s]: specifies the upload period (in seconds) of the port.
      mask Display: port_label('input', 1, PortName)
  visu_MatrixSign_2 : Subsystem  mask(ToSensorWorld){PortName=MatrixSign_2, PortIndex=1, PortWidth=1, TimeStep=1/20}
      mask prompts: PortName "Port Name [-]"; PortIndex "Index [-]"; PortWidth "Port Dimensions [-]"; TimeStep "Upload Period [s]"
      mask help: Sends signal(s) from Simulink to the Sensor World
      mask Help:
      | Sends signal(s) from Simulink to the Sensor World.
      | 
      | - Port Name [-]: specifies the name of the output terminal of the Simulink block.
      | - Index [-]: specifies the start position in the output vector sent to the Sensor World
      | - Port dimensions [-]: specifies the width (number of scalars) of the output port
      | - Upload period [s]: specifies the upload period (in seconds) of the port.
      mask Display: port_label('input', 1, PortName)
  wires:
  SubMuxVisuMatrixSign/1 -> visu_MatrixSign_1/1(Y)
  MatrixSigns/1 -> SubMuxVisuMatrixSign/1
  SubMuxVisuMatrixSign/2 -> visu_MatrixSign_2/1(Y)

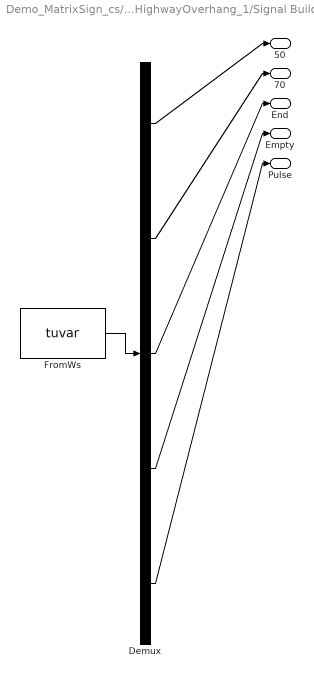
== system Demo_MatrixSign_cs/HighwayOverhang_1/Signal Builder ==
  Demux : Demux  Tag=STV Demux  Outputs=5
  FromWs : FromWorkspace  Tag=STV FromWs  VariableName=tuvar  SampleTime=0  SigBuilderData=DataTag1  VnvData=DataTag2
      SigBuilderData=|
      | common.afterFinalStr = 'Extrapolate'
      | common.sampleTime = 0
      | dataSet.timeRange = [0 10]
      | dataSet.name = 'Group 1'
      | sbobj.Groups.Name = 'Group 1'
      | sbobj.Groups.Signals(1).Name = '50'
      | sbobj.Groups.Signals(1).XData = [0 4 4 7 7 10]
      | sbobj.Groups.Signals(1).YData = [0 0 1 1 0 0]
      | sbobj.Groups.Signals(2).Name = '70'
      | sbobj.Groups.Signals(2).XData = [0 1 1 4 4 10]
      | sbobj.Groups.Signals(2).YData = [0 0 2 2 0 0]
      | sbobj.Groups.Signals(3).Name = 'End'
      | sbobj.Groups.Signals(3).XData = [0 7 7 9 9 10]
      | sbobj.Groups.Signals(3).YData = [0 0 3 3 0 0]
      | sbobj.Groups.Signals(4).Name = 'Empty'
      | sbobj.Groups.Signals(4).XData = [0 1 1 9 9 10]
      | sbobj.Groups.Signals(4).YData = [4 4 0 0 4 4]
      | sbobj.Groups.Signals(5).Name = 'Pulse'
      | sbobj.Groups.Signals(5).XData = [0 1 1 2 2 4 4 5 5 10]
      | sbobj.Groups.Signals(5).YData = [0 0 1 1 0 0 1 1 0 0]
  50 : Outport  Tag=STV Outport
  70 : Outport  Tag=STV Outport  Port=2
  End : Outport  Tag=STV Outport  Port=3
  Empty : Outport  Tag=STV Outport  Port=4
  Pulse : Outport  Tag=STV Outport  Port=5
  wires:
  FromWs/1 -> Demux/1
  Demux/1 -> 50/1
  Demux/2 -> 70/1
  Demux/3 -> End/1
  Demux/4 -> Empty/1
  Demux/5 -> Pulse/1

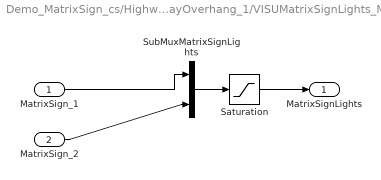
== system Demo_MatrixSign_cs/HighwayOverhang_1/VISUMatrixSignLights_Mux ==
  MatrixSign_1 : Inport  PortDimensions=4
  MatrixSign_2 : Inport  Port=2  PortDimensions=4
  Saturation : Saturate  UpperLimit=1  LowerLimit=0
  SubMuxMatrixSignLights : Mux  Inputs=2
  MatrixSignLights : Outport
  wires:
  SubMuxMatrixSignLights/1 -> Saturation/1
  MatrixSign_1/1 -> SubMuxMatrixSignLights/1
  Saturation/1 -> MatrixSignLights/1
  MatrixSign_2/1 -> SubMuxMatrixSignLights/2

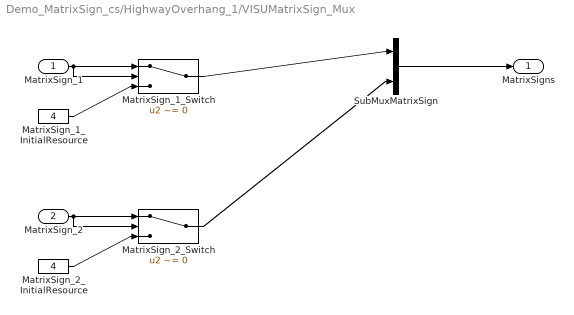
== system Demo_MatrixSign_cs/HighwayOverhang_1/VISUMatrixSign_Mux ==
  MatrixSign_1 : Inport
  MatrixSign_2 : Inport  Port=2
  MatrixSign_1_InitialResource : Constant  Value=4
  MatrixSign_1_Switch : Switch  Criteria=u2 ~= 0
  MatrixSign_2_InitialResource : Constant  Value=4
  MatrixSign_2_Switch : Switch  Criteria=u2 ~= 0
  SubMuxMatrixSign : Mux  Inputs=2
  MatrixSigns : Outport
  wires:
  SubMuxMatrixSign/1 -> MatrixSigns/1
  MatrixSign_1/1 -> MatrixSign_1_Switch/1, MatrixSign_1_Switch/2
  MatrixSign_1_InitialResource/1 -> MatrixSign_1_Switch/3
  MatrixSign_1_Switch/1 -> SubMuxMatrixSign/1
  MatrixSign_2/1 -> MatrixSign_2_Switch/1, MatrixSign_2_Switch/2
  MatrixSign_2_InitialResource/1 -> MatrixSign_2_Switch/3
  MatrixSign_2_Switch/1 -> SubMuxMatrixSign/2

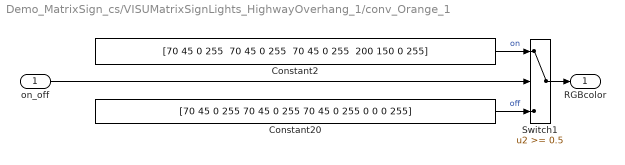
== system Demo_MatrixSign_cs/VISUMatrixSignLights_HighwayOverhang_1/conv_Orange_1 ==
  on_off : Inport
  Constant2 : Constant  Value="[70 45 0 255  70 45 0 255  70 45 0 255  200 150 0 255]"
  Constant20 : Constant  Value=[70 45 0 255 70 45 0 255 70 45 0 255 0 0 0 255]
  Switch1 : Switch  Threshold=0.5
  RGBcolor : Outport
  wires:
  Constant20/1 -> Switch1/3  "off"
  Constant2/1 -> Switch1/1  "on"
  on_off/1 -> Switch1/2
  Switch1/1 -> RGBcolor/1

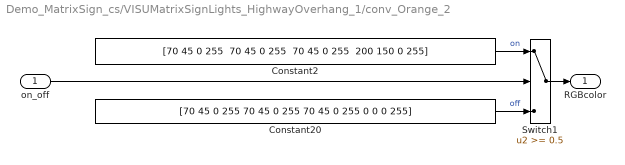
== system Demo_MatrixSign_cs/VISUMatrixSignLights_HighwayOverhang_1/conv_Orange_2 ==
  on_off : Inport
  Constant2 : Constant  Value="[70 45 0 255  70 45 0 255  70 45 0 255  200 150 0 255]"
  Constant20 : Constant  Value=[70 45 0 255 70 45 0 255 70 45 0 255 0 0 0 255]
  Switch1 : Switch  Threshold=0.5
  RGBcolor : Outport
  wires:
  Switch1/1 -> RGBcolor/1
  on_off/1 -> Switch1/2
  Constant2/1 -> Switch1/1  "on"
  Constant20/1 -> Switch1/3  "off"

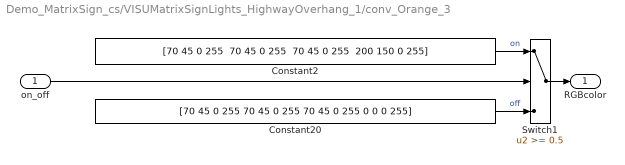
== system Demo_MatrixSign_cs/VISUMatrixSignLights_HighwayOverhang_1/conv_Orange_3 ==
  on_off : Inport
  Constant2 : Constant  Value="[70 45 0 255  70 45 0 255  70 45 0 255  200 150 0 255]"
  Constant20 : Constant  Value=[70 45 0 255 70 45 0 255 70 45 0 255 0 0 0 255]
  Switch1 : Switch  Threshold=0.5
  RGBcolor : Outport
  wires:
  Switch1/1 -> RGBcolor/1
  on_off/1 -> Switch1/2
  Constant2/1 -> Switch1/1  "on"
  Constant20/1 -> Switch1/3  "off"

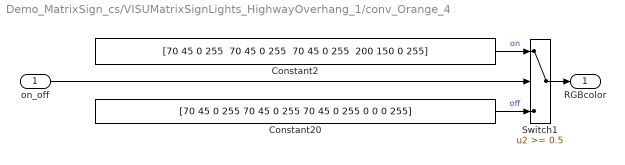
== system Demo_MatrixSign_cs/VISUMatrixSignLights_HighwayOverhang_1/conv_Orange_4 ==
  on_off : Inport
  Constant2 : Constant  Value="[70 45 0 255  70 45 0 255  70 45 0 255  200 150 0 255]"
  Constant20 : Constant  Value=[70 45 0 255 70 45 0 255 70 45 0 255 0 0 0 255]
  Switch1 : Switch  Threshold=0.5
  RGBcolor : Outport
  wires:
  Switch1/1 -> RGBcolor/1
  on_off/1 -> Switch1/2
  Constant2/1 -> Switch1/1  "on"
  Constant20/1 -> Switch1/3  "off"

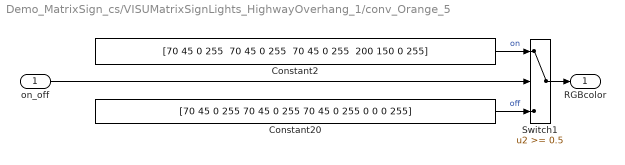
== system Demo_MatrixSign_cs/VISUMatrixSignLights_HighwayOverhang_1/conv_Orange_5 ==
  on_off : Inport
  Constant2 : Constant  Value="[70 45 0 255  70 45 0 255  70 45 0 255  200 150 0 255]"
  Constant20 : Constant  Value=[70 45 0 255 70 45 0 255 70 45 0 255 0 0 0 255]
  Switch1 : Switch  Threshold=0.5
  RGBcolor : Outport
  wires:
  Switch1/1 -> RGBcolor/1
  on_off/1 -> Switch1/2
  Constant2/1 -> Switch1/1  "on"
  Constant20/1 -> Switch1/3  "off"

== system Demo_MatrixSign_cs/VISUMatrixSignLights_HighwayOverhang_1/conv_Orange_6 ==
  on_off : Inport
  Constant2 : Constant  Value="[70 45 0 255  70 45 0 255  70 45 0 255  200 150 0 255]"
  Constant20 : Constant  Value=[70 45 0 255 70 45 0 255 70 45 0 255 0 0 0 255]
  Switch1 : Switch  Threshold=0.5
  RGBcolor : Outport
  wires:
  Switch1/1 -> RGBcolor/1
  on_off/1 -> Switch1/2
  Constant2/1 -> Switch1/1  "on"
  Constant20/1 -> Switch1/3  "off"

== system Demo_MatrixSign_cs/VISUMatrixSignLights_HighwayOverhang_1/conv_Orange_7 ==
  on_off : Inport
  Constant2 : Constant  Value="[70 45 0 255  70 45 0 255  70 45 0 255  200 150 0 255]"
  Constant20 : Constant  Value=[70 45 0 255 70 45 0 255 70 45 0 255 0 0 0 255]
  Switch1 : Switch  Threshold=0.5
  RGBcolor : Outport
  wires:
  Switch1/1 -> RGBcolor/1
  on_off/1 -> Switch1/2
  Constant2/1 -> Switch1/1  "on"
  Constant20/1 -> Switch1/3  "off"

== system Demo_MatrixSign_cs/VISUMatrixSignLights_HighwayOverhang_1/conv_Orange_8 ==
  on_off : Inport
  Constant2 : Constant  Value="[70 45 0 255  70 45 0 255  70 45 0 255  200 150 0 255]"
  Constant20 : Constant  Value=[70 45 0 255 70 45 0 255 70 45 0 255 0 0 0 255]
  Switch1 : Switch  Threshold=0.5
  RGBcolor : Outport
  wires:
  Switch1/1 -> RGBcolor/1
  on_off/1 -> Switch1/2
  Constant2/1 -> Switch1/1  "on"
  Constant20/1 -> Switch1/3  "off"

== system Demo_MatrixSign_cs/VISUMatrixSignLights_HighwayOverhang_1/visu_MatrixSignLights_1 ==
  Y : Inport
  Assignment : Assignment  IndexMode=Zero-based  SampleTime=TimeStep  IndexOptions=Starting index (dialog)  Indices=PortIndex  OutputSizes=[1 1]
  Data Store Read : DataStoreRead  DataStoreName=SimCoreActuators  SampleTime=TimeStep
  Data Store Write : DataStoreWrite  DataStoreName=SimCoreActuators
  wires:
  Y/1 -> Assignment/2
  Data Store Read/1 -> Assignment/1
  Assignment/1 -> Data Store Write/1

== system Demo_MatrixSign_cs/VISUMatrixSignLights_HighwayOverhang_1/visu_MatrixSignLights_2 ==
  Y : Inport
  Assignment : Assignment  IndexMode=Zero-based  SampleTime=TimeStep  IndexOptions=Starting index (dialog)  Indices=PortIndex  OutputSizes=[1 1]
  Data Store Read : DataStoreRead  DataStoreName=SimCoreActuators  SampleTime=TimeStep
  Data Store Write : DataStoreWrite  DataStoreName=SimCoreActuators
  wires:
  Assignment/1 -> Data Store Write/1
  Data Store Read/1 -> Assignment/1
  Y/1 -> Assignment/2

== system Demo_MatrixSign_cs/VISUMatrixSignLights_HighwayOverhang_1/visu_MatrixSignLights_3 ==
  Y : Inport
  Assignment : Assignment  IndexMode=Zero-based  SampleTime=TimeStep  IndexOptions=Starting index (dialog)  Indices=PortIndex  OutputSizes=[1 1]
  Data Store Read : DataStoreRead  DataStoreName=SimCoreActuators  SampleTime=TimeStep
  Data Store Write : DataStoreWrite  DataStoreName=SimCoreActuators
  wires:
  Assignment/1 -> Data Store Write/1
  Data Store Read/1 -> Assignment/1
  Y/1 -> Assignment/2

== system Demo_MatrixSign_cs/VISUMatrixSignLights_HighwayOverhang_1/visu_MatrixSignLights_4 ==
  Y : Inport
  Assignment : Assignment  IndexMode=Zero-based  SampleTime=TimeStep  IndexOptions=Starting index (dialog)  Indices=PortIndex  OutputSizes=[1 1]
  Data Store Read : DataStoreRead  DataStoreName=SimCoreActuators  SampleTime=TimeStep
  Data Store Write : DataStoreWrite  DataStoreName=SimCoreActuators
  wires:
  Assignment/1 -> Data Store Write/1
  Data Store Read/1 -> Assignment/1
  Y/1 -> Assignment/2

== system Demo_MatrixSign_cs/VISUMatrixSignLights_HighwayOverhang_1/visu_MatrixSignLights_5 ==
  Y : Inport
  Assignment : Assignment  IndexMode=Zero-based  SampleTime=TimeStep  IndexOptions=Starting index (dialog)  Indices=PortIndex  OutputSizes=[1 1]
  Data Store Read : DataStoreRead  DataStoreName=SimCoreActuators  SampleTime=TimeStep
  Data Store Write : DataStoreWrite  DataStoreName=SimCoreActuators
  wires:
  Assignment/1 -> Data Store Write/1
  Data Store Read/1 -> Assignment/1
  Y/1 -> Assignment/2

== system Demo_MatrixSign_cs/VISUMatrixSignLights_HighwayOverhang_1/visu_MatrixSignLights_6 ==
  Y : Inport
  Assignment : Assignment  IndexMode=Zero-based  SampleTime=TimeStep  IndexOptions=Starting index (dialog)  Indices=PortIndex  OutputSizes=[1 1]
  Data Store Read : DataStoreRead  DataStoreName=SimCoreActuators  SampleTime=TimeStep
  Data Store Write : DataStoreWrite  DataStoreName=SimCoreActuators
  wires:
  Assignment/1 -> Data Store Write/1
  Data Store Read/1 -> Assignment/1
  Y/1 -> Assignment/2

== system Demo_MatrixSign_cs/VISUMatrixSignLights_HighwayOverhang_1/visu_MatrixSignLights_7 ==
  Y : Inport
  Assignment : Assignment  IndexMode=Zero-based  SampleTime=TimeStep  IndexOptions=Starting index (dialog)  Indices=PortIndex  OutputSizes=[1 1]
  Data Store Read : DataStoreRead  DataStoreName=SimCoreActuators  SampleTime=TimeStep
  Data Store Write : DataStoreWrite  DataStoreName=SimCoreActuators
  wires:
  Assignment/1 -> Data Store Write/1
  Data Store Read/1 -> Assignment/1
  Y/1 -> Assignment/2

== system Demo_MatrixSign_cs/VISUMatrixSignLights_HighwayOverhang_1/visu_MatrixSignLights_8 ==
  Y : Inport
  Assignment : Assignment  IndexMode=Zero-based  SampleTime=TimeStep  IndexOptions=Starting index (dialog)  Indices=PortIndex  OutputSizes=[1 1]
  Data Store Read : DataStoreRead  DataStoreName=SimCoreActuators  SampleTime=TimeStep
  Data Store Write : DataStoreWrite  DataStoreName=SimCoreActuators
  wires:
  Assignment/1 -> Data Store Write/1
  Data Store Read/1 -> Assignment/1
  Y/1 -> Assignment/2

== system Demo_MatrixSign_cs/VISUMatrixSign_HighwayOverhang_1/visu_MatrixSign_1 ==
  Y : Inport
  Assignment : Assignment  IndexMode=Zero-based  SampleTime=TimeStep  IndexOptions=Starting index (dialog)  Indices=PortIndex  OutputSizes=[1 1]
  Data Store Read : DataStoreRead  DataStoreName=SimCoreActuators  SampleTime=TimeStep
  Data Store Write : DataStoreWrite  DataStoreName=SimCoreActuators
  wires:
  Assignment/1 -> Data Store Write/1
  Data Store Read/1 -> Assignment/1
  Y/1 -> Assignment/2

== system Demo_MatrixSign_cs/VISUMatrixSign_HighwayOverhang_1/visu_MatrixSign_2 ==
  Y : Inport
  Assignment : Assignment  IndexMode=Zero-based  SampleTime=TimeStep  IndexOptions=Starting index (dialog)  Indices=PortIndex  OutputSizes=[1 1]
  Data Store Read : DataStoreRead  DataStoreName=SimCoreActuators  SampleTime=TimeStep
  Data Store Write : DataStoreWrite  DataStoreName=SimCoreActuators
  wires:
  Y/1 -> Assignment/2
  Data Store Read/1 -> Assignment/1
  Assignment/1 -> Data Store Write/1
